simulink library "STMM"  (R2024a)
settings: Solver=VariableStepAuto  StartTime=0.0  StopTime=10.0  RelTol=1e-3
undefined symbols (not defined in the file): raptor_xcp_function, StateCAN
libraries: Utilities x130, Raptor_lib x34, simulink x1
(part 1 of 2)
settings Model: Creator=serga  LastModifiedBy=serga

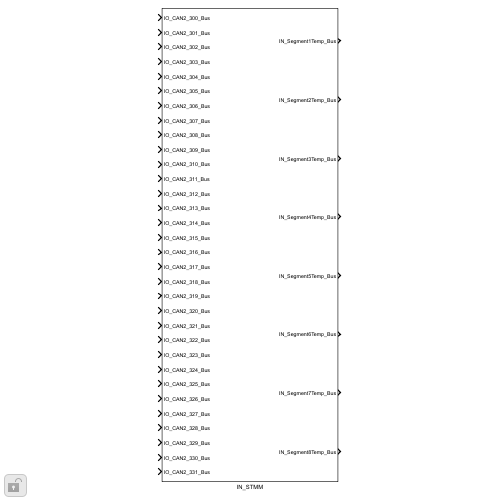
[thumbnail: Simulink's stored preview of the top-level diagram]
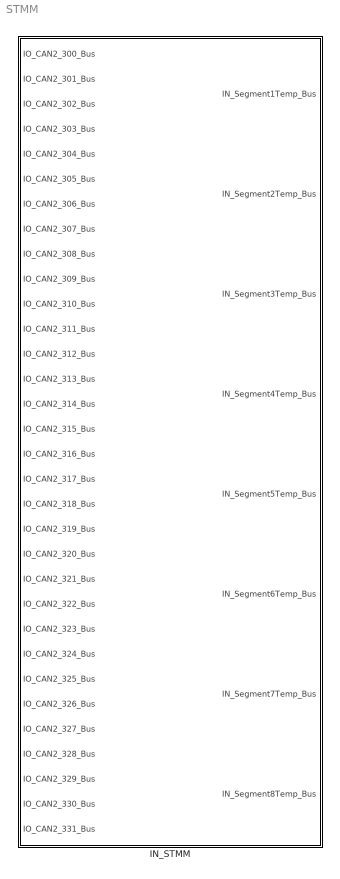
== system STMM ==
  IN_STMM : Subsystem
